simulink model "lab_4_4_bpsk_ideal_ber_awgn"  (R2025a)
settings: Solver=FixedStepDiscrete  StartTime=0.0  StopTime=lab44_ber_stop_time  FixedStep=1  RelTol=1e-3
InitFcn:
  | lab_4_4_ensure_bpsk_simulink_workspace;
undefined symbols (not defined in the file): lab44_ber_noise_sigma
libraries: simulink x1
settings Model: Creator=user  LastModifiedBy=user

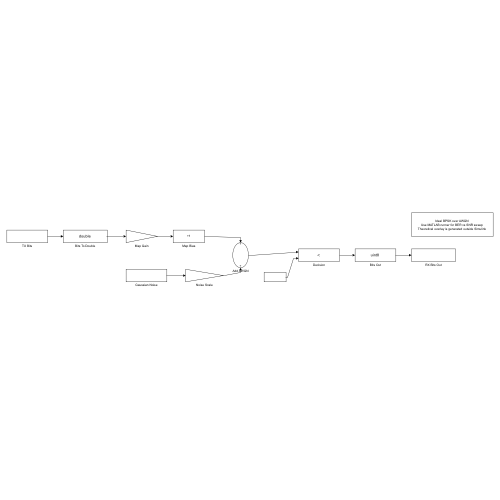
[thumbnail: Simulink's stored preview of the top-level diagram]
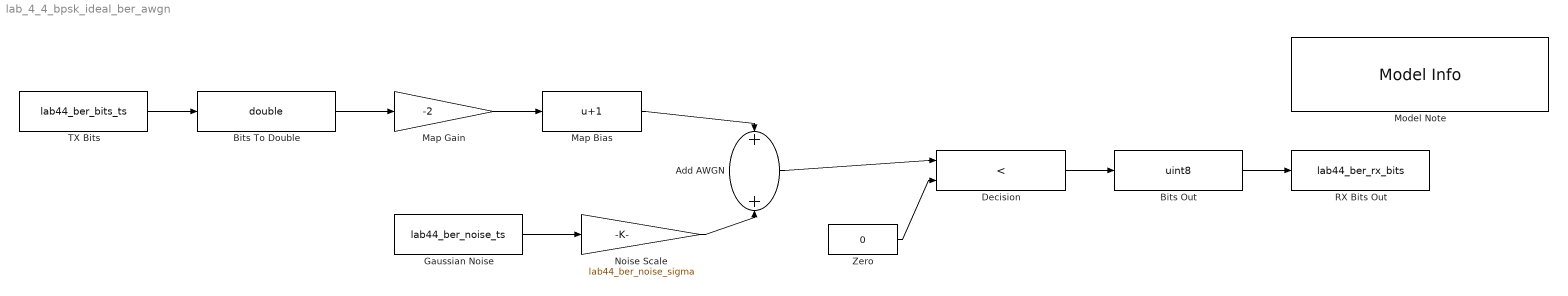
== system lab_4_4_bpsk_ideal_ber_awgn ==
  Add AWGN : Sum
  Bits Out : DataTypeConversion  OutDataTypeStr=uint8  SaturateOnIntegerOverflow=off  RndMeth=Floor
  Bits To Double : DataTypeConversion  OutDataTypeStr=double  SaturateOnIntegerOverflow=off  RndMeth=Floor
  Decision : RelationalOperator  Operator=<  OutDataTypeStr=boolean  RndMeth=Simplest  InputSameDT=off
  Gaussian Noise : FromWorkspace  VariableName=lab44_ber_noise_ts
  Map Bias : Bias  Bias=1  SaturateOnIntegerOverflow=off
  Map Gain : Gain  Gain=-2
  Model Note : simulink/Model-Wide Utilities/Model Info  Frame=on  DisplayStringWithTags=Model Info  HorizontalTextAlignment=Center  LeftAlignmentValue=0.5
  Noise Scale : Gain  Gain=lab44_ber_noise_sigma
  RX Bits Out : ToWorkspace  VariableName=lab44_ber_rx_bits  SaveFormat=Timeseries  SampleTime=-1
  TX Bits : FromWorkspace  VariableName=lab44_ber_bits_ts
  Zero : Constant  Value=0
  wires:
  TX Bits/1 -> Bits To Double/1
  Bits To Double/1 -> Map Gain/1
  Map Gain/1 -> Map Bias/1
  Map Bias/1 -> Add AWGN/1
  Gaussian Noise/1 -> Noise Scale/1
  Noise Scale/1 -> Add AWGN/2
  Add AWGN/1 -> Decision/1
  Zero/1 -> Decision/2
  Decision/1 -> Bits Out/1
  Bits Out/1 -> RX Bits Out/1
